simulink model "Zeta_Conv"  (R2024a)
settings: Solver=VariableStepAuto  StartTime=0.0  StopTime=10  RelTol=1e-3
libraries: spsSeriesRLCBranchLib x10, spsVoltageMeasurementLib x6, spsMeanLib x4, spsCurrentMeasurementLib x2, spsDCVoltageSourceLib x2, spsDiodeLib x2, spsGroundLib x2, spsMosfetLib x2, spsPWMGeneratorDCDCLib x2, sps_lib x1
settings Model: Creator=Varad  LastModifiedBy=Varad

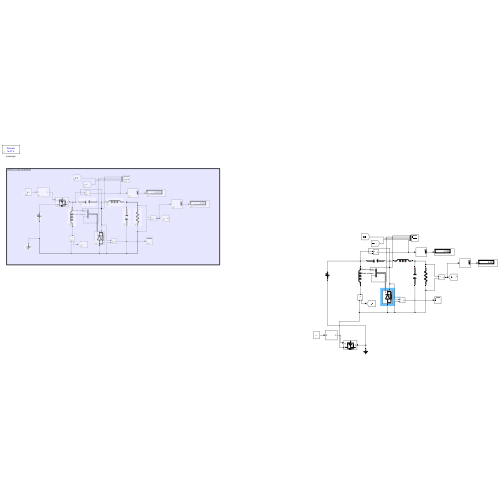
[thumbnail: Simulink's stored preview of the top-level diagram]
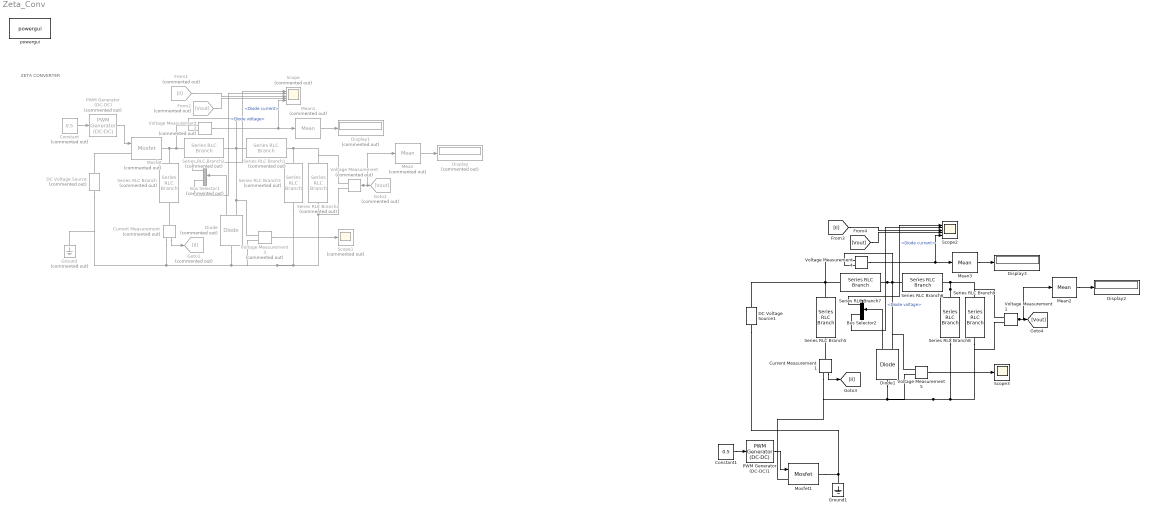
== system Zeta_Conv ==
  note: ZETA CONVERTER
  Bus Selector1 : BusSelector  Commented=on  OutputSignals=Diode current,Diode voltage
  Bus Selector2 : BusSelector  OutputSignals=Diode current,Diode voltage
  Constant : Constant  Commented=on  Value=0.5
  Constant1 : Constant  Value=0.5
  Current Measurement : spsCurrentMeasurementLib/Current Measurement  Commented=on  PhasorSimulation=off  OutputType=Complex  PSBequivalent=0
  Current Measurement1 : spsCurrentMeasurementLib/Current Measurement  PhasorSimulation=off  OutputType=Complex  PSBequivalent=0
  DC Voltage Source : spsDCVoltageSourceLib/DC Voltage Source  Commented=on  Amplitude=4  Measurements=None
  DC Voltage Source1 : spsDCVoltageSourceLib/DC Voltage Source  Amplitude=4  Measurements=None
  Diode : spsDiodeLib/Diode  Commented=on  Ron=1e-7  Lon=0  Vf=0.8  IC=0  UseSnubber=0  Rs=1e6  Cs=1e6  Measurements=on
  Diode1 : spsDiodeLib/Diode  Ron=1e-7  Lon=0  Vf=0  IC=0  UseSnubber=0  Rs=1e6  Cs=1e6  Measurements=on
  Display : Display  Commented=on
  Display1 : Display  Commented=on
  Display2 : Display
  Display3 : Display
  From1 : From  Commented=on  GotoTag=Il
  From2 : From  Commented=on  GotoTag=Vout
  Goto1 : Goto  Commented=on  GotoTag=Il
  Goto2 : Goto  Commented=on  GotoTag=Vout
  Ground : spsGroundLib/Ground  Commented=on  LConnTagsString=a
  Ground1 : spsGroundLib/Ground  LConnTagsString=a
  Mean : spsMeanLib/Mean  Commented=on  Freq=60  Vinit=0  Ts=0
  Mean1 : spsMeanLib/Mean  Commented=on  Freq=60  Vinit=0  Ts=0
  Mean2 : spsMeanLib/Mean  Freq=60  Vinit=0  Ts=0
  Mean3 : spsMeanLib/Mean  Freq=60  Vinit=0  Ts=0
  Mosfet : spsMosfetLib/Mosfet  Commented=on  Ron=1e-7  Lon=0  Rd=1e-10  Vfd=0  IC=0  Rs=inf  Cs=0  Measurements=off
  Mosfet1 : spsMosfetLib/Mosfet  Ron=1e-7  Lon=0  Rd=1e-10  Vfd=0  IC=0  Rs=inf  Cs=0  Measurements=off
  PWM Generator (DC-DC) : spsPWMGeneratorDCDCLib/PWM Generator (DC-DC)  Commented=on  Fsw=15000  Ts=1e-7
  PWM Generator (DC-DC)1 : spsPWMGeneratorDCDCLib/PWM Generator (DC-DC)  Fsw=15000  Ts=1e-7
  Scope : Scope  Commented=on  NumInputPorts=5
  Scope1 : Scope  Commented=on
  Scope2 : Scope  NumInputPorts=5
  Scope3 : Scope
  Series RLC Branch : spsSeriesRLCBranchLib/Series RLC Branch  Commented=on  LConnTagsString=__new0  RConnTagsString=__new0  BranchType=L  Resistance=1  Inductance=1e-3  SetiL0=off  InitialCurrent=0  Capacitance=1e-6  Setx0=off  InitialVoltage=0  Measurements=None
  Series RLC Branch1 : spsSeriesRLCBranchLib/Series RLC Branch  Commented=on  LConnTagsString=__new0  RConnTagsString=__new0  BranchType=L  Resistance=1  Inductance=1e-3  SetiL0=off  InitialCurrent=0  Capacitance=1e-6  Setx0=off  InitialVoltage=0  Measurements=None
  Series RLC Branch2 : spsSeriesRLCBranchLib/Series RLC Branch  Commented=on  LConnTagsString=__new0  RConnTagsString=__new0  BranchType=C  Resistance=1  Inductance=1e-3  SetiL0=off  InitialCurrent=0  Capacitance=200e-6  Setx0=off  InitialVoltage=12  Measurements=None
  Series RLC Branch3 : spsSeriesRLCBranchLib/Series RLC Branch  Commented=on  LConnTagsString=__new0  RConnTagsString=__new0  BranchType=C  Resistance=1  Inductance=1e-3  SetiL0=off  InitialCurrent=0  Capacitance=470e-6  Setx0=off  InitialVoltage=12  Measurements=None
  Series RLC Branch4 : spsSeriesRLCBranchLib/Series RLC Branch  Commented=on  LConnTagsString=__new0  RConnTagsString=__new0  BranchType=R  Resistance=10  Inductance=1e-3  SetiL0=off  InitialCurrent=0  Capacitance=1e-6  Setx0=off  InitialVoltage=0  Measurements=None
  Series RLC Branch5 : spsSeriesRLCBranchLib/Series RLC Branch  LConnTagsString=__new0  RConnTagsString=__new0  BranchType=L  Resistance=1  Inductance=1e-3  SetiL0=off  InitialCurrent=0  Capacitance=1e-6  Setx0=off  InitialVoltage=0  Measurements=None
  Series RLC Branch6 : spsSeriesRLCBranchLib/Series RLC Branch  LConnTagsString=__new0  RConnTagsString=__new0  BranchType=L  Resistance=1  Inductance=1e-3  SetiL0=off  InitialCurrent=0  Capacitance=1e-6  Setx0=off  InitialVoltage=0  Measurements=None
  Series RLC Branch7 : spsSeriesRLCBranchLib/Series RLC Branch  LConnTagsString=__new0  RConnTagsString=__new0  BranchType=C  Resistance=1  Inductance=1e-3  SetiL0=off  InitialCurrent=0  Capacitance=200e-6  Setx0=off  InitialVoltage=12  Measurements=None
  Series RLC Branch8 : spsSeriesRLCBranchLib/Series RLC Branch  LConnTagsString=__new0  RConnTagsString=__new0  BranchType=C  Resistance=1  Inductance=1e-3  SetiL0=off  InitialCurrent=0  Capacitance=50e-6  Setx0=off  InitialVoltage=12  Measurements=None
  Series RLC Branch9 : spsSeriesRLCBranchLib/Series RLC Branch  LConnTagsString=__new0  RConnTagsString=__new0  BranchType=R  Resistance=10  Inductance=1e-3  SetiL0=off  InitialCurrent=0  Capacitance=1e-6  Setx0=off  InitialVoltage=0  Measurements=None
  Voltage Measurement : spsVoltageMeasurementLib/Voltage Measurement  Commented=on  PhasorSimulation=off  OutputType=Complex  PSBequivalent=0
  Voltage Measurement1 : spsVoltageMeasurementLib/Voltage Measurement  PhasorSimulation=off  OutputType=Complex  PSBequivalent=0
  Voltage Measurement2 : spsVoltageMeasurementLib/Voltage Measurement  Commented=on  PhasorSimulation=off  OutputType=Complex  PSBequivalent=0
  Voltage Measurement3 : spsVoltageMeasurementLib/Voltage Measurement  Commented=on  PhasorSimulation=off  OutputType=Complex  PSBequivalent=0
  Voltage Measurement4 : spsVoltageMeasurementLib/Voltage Measurement  PhasorSimulation=off  OutputType=Complex  PSBequivalent=0
  Voltage Measurement5 : spsVoltageMeasurementLib/Voltage Measurement  PhasorSimulation=off  OutputType=Complex  PSBequivalent=0
  powergui : sps_lib/powergui  Priority=1  SimulationMode=Discrete  SampleTime=1e-7  frequency=60  Iterations=50  frequencyindice=0  Pbase=100e6  ErrMax=1e-4  UnitsV=kV  UnitsW=MW  buscounter=0  FunctionMessages=off  echomessages=off  EnableUseOfTLC=off  CurrentSourceSwitches=off  DisableSnubberDevices=off  DisableRonSwitches=off  DisableVfSwitches=off  DisplayEquations=off  AutomaticDiscreteSolvers=off  SolverType=Tustin/Backward Euler (TBE)  Interpol=off  ExternalGateDelay=off  methode=off  Ts=100  x0status=blocks  SPID=on  SwTol=0  HookPort=off  NonlinearTolerance=1e-4  nMaxIteration=100  ContinueOnMaxIteration=off  RestoreLinks=warning  ResistiveCurrentMeasurement=off  Frange=[0:2:500]  Ylog=off  Xlog=on  ShowGrid=off  save=off  variable=ZData  structure=0  ZoomFFT=off  StartTime=0.0  cycles=1  DisplayStyle=1  fundamental=60  FreqAxis=off  MaxFrequency=1000  frequencyindicesteady=1  RmsSteady=1  display=off
  wires:
  Current Measurement/1 -> Goto1/1
  Constant/1 -> PWM Generator (DC-DC)/1
  PWM Generator (DC-DC)/1 -> Mosfet/1
  Diode/1 -> Bus Selector1/1
  Bus Selector1/1 -> Scope/1  "<Diode current>"
  Bus Selector1/2 -> Scope/2  "<Diode voltage>"
  From1/1 -> Scope/3
  From2/1 -> Scope/4
  Voltage Measurement/1 -> Mean/1, Goto2/1
  Mean/1 -> Display/1
  Mean1/1 -> Display1/1
  Voltage Measurement2/1 -> Mean1/1, Scope/5
  Voltage Measurement3/1 -> Scope1/1
  Voltage Measurement5/1 -> Scope3/1
  Bus Selector2/2 -> Scope2/2  "<Diode voltage>"
  Voltage Measurement4/1 -> Mean3/1, Scope2/5
  Mean2/1 -> Display2/1
  Diode1/1 -> Bus Selector2/1
  [Vout] -> Scope2/4
  PWM Generator (DC-DC)1/1 -> Mosfet1/1
  Bus Selector2/1 -> Scope2/1  "<Diode current>"
  [Il] -> Scope2/3
  Constant1/1 -> PWM Generator (DC-DC)1/1
  Mean3/1 -> Display3/1
  Current Measurement1/1 -> [Il]
  Voltage Measurement1/1 -> Mean2/1, [Vout]
  connections:
  DC Voltage Source/RConn1 -- Mosfet/LConn1
  Series RLC Branch/LConn1 -- Voltage Measurement2/LConn1 -- Series RLC Branch2/LConn1 -- Mosfet/RConn1
  Diode/RConn1 -- Voltage Measurement3/LConn1 -- Voltage Measurement2/LConn2 -- Series RLC Branch1/LConn1 -- Series RLC Branch2/RConn1
  Series RLC Branch1/RConn1 -- Voltage Measurement/LConn1 -- Series RLC Branch4/LConn1 -- Series RLC Branch3/LConn1
  Current Measurement/LConn1 -- Series RLC Branch/RConn1
  Voltage Measurement/LConn2 -- Series RLC Branch4/RConn1 -- Voltage Measurement3/LConn2 -- Ground/LConn1 -- DC Voltage Source/LConn1 -- Current Measurement/RConn1 -- Diode/LConn1 -- Series RLC Branch3/RConn1
  Series RLC Branch7/RConn1 -- Voltage Measurement5/LConn1 -- Diode1/RConn1 -- Voltage Measurement4/LConn2 -- Series RLC Branch6/LConn1
  Diode1/LConn1 -- Mosfet1/LConn1 -- Current Measurement1/RConn1 -- Voltage Measurement5/LConn2 -- Voltage Measurement1/LConn2 -- Series RLC Branch9/RConn1 -- Series RLC Branch8/RConn1
  Series RLC Branch8/LConn1 -- Series RLC Branch6/RConn1 -- Voltage Measurement1/LConn1 -- Series RLC Branch9/LConn1
  Series RLC Branch7/LConn1 -- Voltage Measurement4/LConn1 -- DC Voltage Source1/RConn1 -- Series RLC Branch5/LConn1
  Current Measurement1/LConn1 -- Series RLC Branch5/RConn1
  Mosfet1/RConn1 -- DC Voltage Source1/LConn1 -- Ground1/LConn1
